simulink model "dsp_channelized_receiver_"  (R2021a)
settings: Solver=VariableStepAuto  StartTime=0.0  StopTime=sim_time  RelTol=1e-3
values from neighbouring files (symbols this model uses):
  sim_time = 1e-3    (= 0.001)    [rx_dsp_core_init_hw.m]
  ts = 1/fs    (= 2.5e-10)    [rx_dsp_core_init_hw.m]
undefined symbols (not defined in the file or in its folder): es1
libraries: xbsIndex_r4 x267, dspsrcs4 x3, simulink x1, dspswit3 x1
(part 2 of 2)

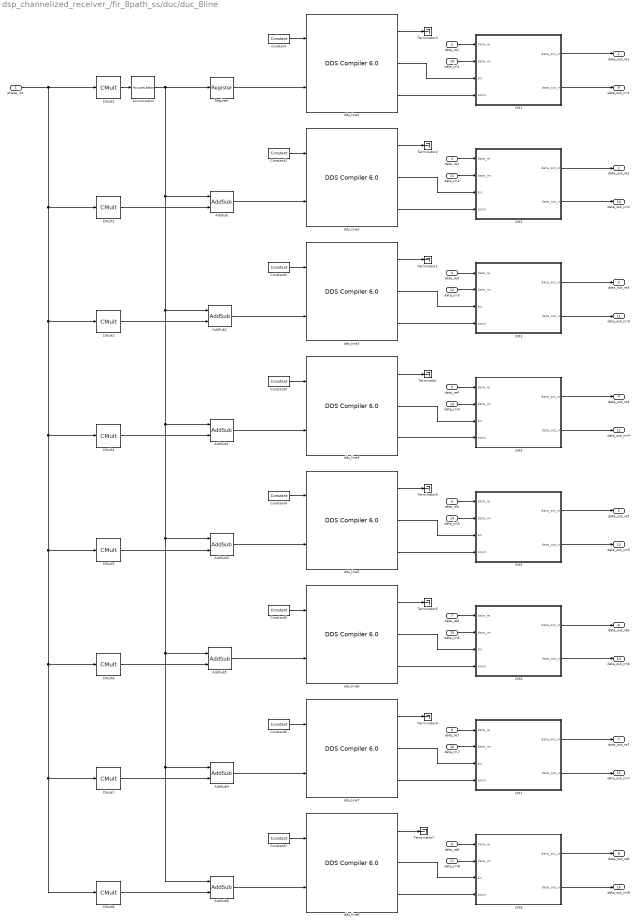
== system dsp_channelized_receiver_/fir_8path_ss/duc/duc_8line ==
  phase_inc : Inport
  data_re1 : Inport  Port=2
  data_re2 : Inport  Port=3
  data_re3 : Inport  Port=4
  data_re4 : Inport  Port=5
  data_re5 : Inport  Port=6
  data_re6 : Inport  Port=7
  data_re7 : Inport  Port=8
  data_re8 : Inport  Port=9
  data_im1 : Inport  Port=10
  data_im2 : Inport  Port=11
  data_im3 : Inport  Port=12
  data_im4 : Inport  Port=13
  data_im5 : Inport  Port=14
  data_im6 : Inport  Port=15
  data_im7 : Inport  Port=16
  data_im8 : Inport  Port=17
  Accumulator : xbsIndex_r4/Accumulator  operation=Add  n_bits=ddc_phase_width  overflow=Wrap  scale=1  rst=off  hasbypass=off  infoeditControl=reset for floating point data type must be asserted for a minimum of 2 cycles  en=off  latency=1  msb_inp=100  msb=100  lsb=-100  use_behavioral_HDL=on  implementation=Fabric  dbl_ovrd=off  block_type=accum
  AddSub{,1..6} (7 alike) : xbsIndex_r4/AddSub  mode=Addition  use_carryin=off  use_carryout=off  en=off  latency=1  precision=User Defined  arith_type=Unsigned  n_bits=ddc_phase_width  bin_pt=ddc_phase_width  quantization="Round  (unbiased: +/- Inf)"  overflow=Wrap  use_behavioral_HDL=off  hw_selection=Fabric  pipelined=off  dbl_ovrd=off  block_type=addsub
  CM1 : Subsystem
  CM2 : Subsystem
  CM3 : Subsystem
  CM4 : Subsystem
  CM5 : Subsystem
  CM6 : Subsystem
  CM7 : Subsystem
  CM8 : Subsystem
  CMult1 : xbsIndex_r4/CMult  const=1  gui_display_data_type=Fixed-point  const_n_bits=4  const_bin_pt=0  float_type=Single  exp_bits=8  fraction_bits=24  en=off  latency=1  precision=User Defined  arith_type=Unsigned  n_bits=ddc_phase_width  bin_pt=ddc_phase_width  quantization="Round  (unbiased: +/- Inf)"  overflow=Wrap  use_behavioral_HDL=off  mem_type=Distributed RAM  pipeline=off  dbl_ovrd=off  block_type=cmult
  CMult2 : xbsIndex_r4/CMult  const=2  gui_display_data_type=Fixed-point  const_n_bits=4  const_bin_pt=0  float_type=Single  exp_bits=8  fraction_bits=24  en=off  latency=1  precision=User Defined  arith_type=Unsigned  n_bits=ddc_phase_width  bin_pt=ddc_phase_width  quantization="Round  (unbiased: +/- Inf)"  overflow=Wrap  use_behavioral_HDL=off  mem_type=Distributed RAM  pipeline=off  dbl_ovrd=off  block_type=cmult
  CMult3 : xbsIndex_r4/CMult  const=8  gui_display_data_type=Fixed-point  const_n_bits=4  const_bin_pt=0  float_type=Single  exp_bits=8  fraction_bits=24  en=off  latency=1  precision=User Defined  arith_type=Unsigned  n_bits=ddc_phase_width  bin_pt=ddc_phase_width  quantization="Round  (unbiased: +/- Inf)"  overflow=Wrap  use_behavioral_HDL=off  mem_type=Distributed RAM  pipeline=off  dbl_ovrd=off  block_type=cmult
  CMult4 : xbsIndex_r4/CMult  const=3  gui_display_data_type=Fixed-point  const_n_bits=4  const_bin_pt=0  float_type=Single  exp_bits=8  fraction_bits=24  en=off  latency=1  precision=User Defined  arith_type=Unsigned  n_bits=ddc_phase_width  bin_pt=ddc_phase_width  quantization="Round  (unbiased: +/- Inf)"  overflow=Wrap  use_behavioral_HDL=off  mem_type=Distributed RAM  pipeline=off  dbl_ovrd=off  block_type=cmult
  CMult5 : xbsIndex_r4/CMult  const=4  gui_display_data_type=Fixed-point  const_n_bits=4  const_bin_pt=0  float_type=Single  exp_bits=8  fraction_bits=24  en=off  latency=1  precision=User Defined  arith_type=Unsigned  n_bits=ddc_phase_width  bin_pt=ddc_phase_width  quantization="Round  (unbiased: +/- Inf)"  overflow=Wrap  use_behavioral_HDL=off  mem_type=Distributed RAM  pipeline=off  dbl_ovrd=off  block_type=cmult
  CMult6 : xbsIndex_r4/CMult  const=5  gui_display_data_type=Fixed-point  const_n_bits=4  const_bin_pt=0  float_type=Single  exp_bits=8  fraction_bits=24  en=off  latency=1  precision=User Defined  arith_type=Unsigned  n_bits=ddc_phase_width  bin_pt=ddc_phase_width  quantization="Round  (unbiased: +/- Inf)"  overflow=Wrap  use_behavioral_HDL=off  mem_type=Distributed RAM  pipeline=off  dbl_ovrd=off  block_type=cmult
  CMult7 : xbsIndex_r4/CMult  const=6  gui_display_data_type=Fixed-point  const_n_bits=4  const_bin_pt=0  float_type=Single  exp_bits=8  fraction_bits=24  en=off  latency=1  precision=User Defined  arith_type=Unsigned  n_bits=ddc_phase_width  bin_pt=ddc_phase_width  quantization="Round  (unbiased: +/- Inf)"  overflow=Wrap  use_behavioral_HDL=off  mem_type=Distributed RAM  pipeline=off  dbl_ovrd=off  block_type=cmult
  CMult8 : xbsIndex_r4/CMult  const=7  gui_display_data_type=Fixed-point  const_n_bits=4  const_bin_pt=0  float_type=Single  exp_bits=8  fraction_bits=24  en=off  latency=1  precision=User Defined  arith_type=Unsigned  n_bits=ddc_phase_width  bin_pt=ddc_phase_width  quantization="Round  (unbiased: +/- Inf)"  overflow=Wrap  use_behavioral_HDL=off  mem_type=Distributed RAM  pipeline=off  dbl_ovrd=off  block_type=cmult
  Constant{,1..7} (8 alike) : xbsIndex_r4/Constant  const=1  gui_display_data_type=Boolean  arith_type=Boolean  n_bits=16  bin_pt=14  preci_type=Single  exp_width=8  frac_width=24  explicit_period=on  period=ts  equ=P=C  opselect=C  inp2=PCIN>>17  opr=+  inp1=P  carry=CIN  dbl_ovrd=off  block_type=constant
  Register : xbsIndex_r4/Register  init=0  rst=off  en=off  dbl_ovrd=off  block_type=register
  Terminator{,1..7} (8 alike) : Terminator
  dds_line{1..8} (8 alike) : xbsIndex_r4/DDS Compiler 6.0   partspresent=SIN_COS_LUT_only  dds_clock_rate=100  channels=1  mode_of_operation=Standard  modulus=9  parameter_entry=System_Parameters  spurious_free_dynamic_range=36.00000000  frequency_resolution=0.40000000  noise_shaping=None  phase_width=ddc_phase_width  output_width=ddc_data_width  output_selection=Sine_and_Cosine  negative_sine=off  negative_cosine=off  amplitude_mode=Full_Range  memory_type=Auto  optimization_goal=Auto  dsp48_use=Minimal  resync=off  latency_configuration=Auto  latency=1  has_phase_out=off  has_aclken=off  has_aresetn=off  explicit_period=off  period=1  data_has_tlast=Not_Required  has_tready=off  s_phase_has_tuser=Not_Required  m_data_has_tuser=Not_Required  m_phase_has_tuser=Not_Required  s_phase_tuser_width=1  output_form=Twos_Complement  s_config_sync_mode=On_Vector  phase_increment=Fixed  output_frequency1=0  output_frequency2=0  output_frequency3=0  output_frequency4=0  output_frequency5=0  output_frequency6=0  output_frequency7=0  output_frequency8=0  output_frequency9=0  output_frequency10=0  output_frequency11=0  output_frequency12=0  output_frequency13=0  output_frequency14=0  output_frequency15=0  output_frequency16=0  pinc1='0'  pinc2='0'  pinc3='0'  pinc4='0'  pinc5='0'  pinc6='0'  pinc7='0'  pinc8='0'  pinc9='0'  pinc10='0'  pinc11='0'  pinc12='0'  pinc13='0'  pinc14='0'  pinc15='0'  pinc16='0'  phase_offset=None  phase_offset_angles1=0  phase_offset_angles2=0  phase_offset_angles3=0  phase_offset_angles4=0  phase_offset_angles5=0  phase_offset_angles6=0  phase_offset_angles7=0  phase_offset_angles8=0  phase_offset_angles9=0  phase_offset_angles10=0  phase_offset_angles11=0  phase_offset_angles12=0  phase_offset_angles13=0  phase_offset_angles14=0  phase_offset_angles15=0  phase_offset_angles16=0  poff1='0'  poff2='0'  poff3='0'  poff4='0'  poff5='0'  poff6='0'  poff7='0'  poff8='0'  poff9='0'  poff10='0'  poff11='0'  poff12='0'  poff13='0'  poff14='0'  poff15='0'  poff16='0'  trim_axipin_name=on  simulation_type=hybrid_sim  simulation_model=sysgen:xddsv6_0_cmodel  data_path_portlist={ 's_axis_config_tdata_poff', 's_axis_config_tdata_chan0_poff', 's_axis_config_tdata_pinc', 's_axis_config_tdata_chan0_pinc', 's_axis_phase_tdata_resync', 's_axis_phase_tdata_chan0_resync', 's_axis_phase_tdata_poff', 's_axis_phase_tdata_chan0_poff', 's_axis_phase_tdata_pinc', 's_axis_phase_tdata_chan0_pinc', 's_axis_phase_tdata_phase_in', 'm_axis_data_tdata_sine', 'm_axis_data_tdata_chan0_sine', 'm_axis_data_tdata_cosine', 'm_axis_data_tdata_chan0_cosine', 'm_axis_phase_tdata_phase_out', 'm_axis_phase_tdata_chan0_phase_out'}  por_mode=false  gui_behaviour=Sysgen  ip_name=DDS Compiler  ip_version=6.0  dsptool_ready=true  wrapper_available=true  port_translation_map={ 'aclken' => 'en', 'aresetn' => 'rst' }  ipcore_usecache=true  ipcore_useipmodelcache=true  ipcore_xco_need_fpga_part=true  ipcore_verbose=false  block_type=dds_compiler_v6_0
  data_out_re1 : Outport
  data_out_re2 : Outport  Port=2
  data_out_re3 : Outport  Port=3
  data_out_re4 : Outport  Port=4
  data_out_re5 : Outport  Port=5
  data_out_re6 : Outport  Port=6
  data_out_re7 : Outport  Port=7
  data_out_re8 : Outport  Port=8
  data_out_im1 : Outport  Port=9
  data_out_im2 : Outport  Port=10
  data_out_im3 : Outport  Port=11
  data_out_im4 : Outport  Port=12
  data_out_im5 : Outport  Port=13
  data_out_im6 : Outport  Port=14
  data_out_im7 : Outport  Port=15
  data_out_im8 : Outport  Port=16
  wires:
  Register/1 -> dds_line1/2
  CMult3/1 -> Accumulator/1
  AddSub2/1 -> dds_line3/2
  AddSub1/1 -> dds_line4/2
  AddSub/1 -> dds_line2/2
  dds_line3/1 -> Terminator1/1
  Constant/1 -> dds_line1/1
  dds_line1/1 -> Terminator3/1
  Constant1/1 -> dds_line2/1
  Constant2/1 -> dds_line3/1
  dds_line2/1 -> Terminator2/1
  dds_line4/1 -> Terminator/1
  Constant3/1 -> dds_line4/1
  Constant6/1 -> dds_line7/1
  dds_line7/1 -> Terminator4/1
  dds_line5/1 -> Terminator6/1
  Constant5/1 -> dds_line6/1
  Constant4/1 -> dds_line5/1
  dds_line6/1 -> Terminator5/1
  AddSub3/1 -> dds_line5/2
  AddSub4/1 -> dds_line7/2
  AddSub5/1 -> dds_line6/2
  CMult1/1 -> AddSub/2
  CMult2/1 -> AddSub2/2
  CMult4/1 -> AddSub1/2
  CMult5/1 -> AddSub3/2
  CMult6/1 -> AddSub5/2
  CMult7/1 -> AddSub4/2
  CMult8/1 -> AddSub6/2
  phase_inc/1 -> CMult8/1, CMult7/1, CMult6/1, CMult5/1, CMult4/1, CMult2/1, CMult1/1, CMult3/1
  Accumulator/1 -> AddSub6/1, AddSub4/1, AddSub5/1, AddSub3/1, AddSub1/1, AddSub2/1, AddSub/1, Register/1
  AddSub6/1 -> dds_line8/2
  dds_line8/1 -> Terminator7/1
  Constant7/1 -> dds_line8/1
  dds_line1/3 -> CM1/4(cosin)
  dds_line1/2 -> CM1/3(sin)
  dds_line2/3 -> CM2/4(cosin)
  dds_line3/3 -> CM3/4(cosin)
  dds_line4/3 -> CM4/4(cosin)
  dds_line4/2 -> CM4/3(sin)
  dds_line3/2 -> CM3/3(sin)
  dds_line2/2 -> CM2/3(sin)
  dds_line5/3 -> CM5/4(cosin)
  dds_line5/2 -> CM5/3(sin)
  dds_line6/3 -> CM6/4(cosin)
  dds_line6/2 -> CM6/3(sin)
  dds_line7/3 -> CM7/4(cosin)
  dds_line7/2 -> CM7/3(sin)
  dds_line8/3 -> CM8/4(cosin)
  dds_line8/2 -> CM8/3(sin)
  data_re1/1 -> CM1/1(data_re)
  data_re2/1 -> CM2/1(data_re)
  data_re3/1 -> CM3/1(data_re)
  data_re4/1 -> CM4/1(data_re)
  data_re5/1 -> CM5/1(data_re)
  data_re6/1 -> CM6/1(data_re)
  data_re7/1 -> CM7/1(data_re)
  data_re8/1 -> CM8/1(data_re)
  data_im1/1 -> CM1/2(data_im)
  data_im2/1 -> CM2/2(data_im)
  data_im3/1 -> CM3/2(data_im)
  data_im4/1 -> CM4/2(data_im)
  data_im5/1 -> CM5/2(data_im)
  data_im6/1 -> CM6/2(data_im)
  data_im7/1 -> CM7/2(data_im)
  data_im8/1 -> CM8/2(data_im)
  CM1/1(data_out_im) -> data_out_re1/1
  CM1/2(data_out_re) -> data_out_im1/1
  CM2/2(data_out_re) -> data_out_im2/1
  CM2/1(data_out_im) -> data_out_re2/1
  CM3/2(data_out_re) -> data_out_im3/1
  CM3/1(data_out_im) -> data_out_re3/1
  CM4/2(data_out_re) -> data_out_im4/1
  CM4/1(data_out_im) -> data_out_re4/1
  CM5/2(data_out_re) -> data_out_im5/1
  CM5/1(data_out_im) -> data_out_re5/1
  CM6/2(data_out_re) -> data_out_im6/1
  CM6/1(data_out_im) -> data_out_re6/1
  CM7/2(data_out_re) -> data_out_im7/1
  CM7/1(data_out_im) -> data_out_re7/1
  CM8/2(data_out_re) -> data_out_im8/1
  CM8/1(data_out_im) -> data_out_re8/1

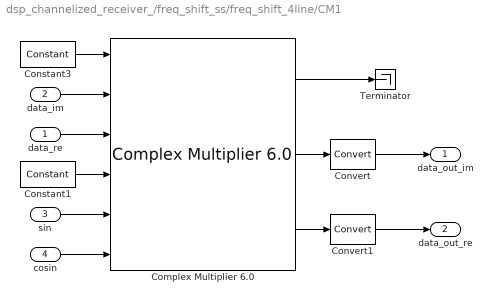
== system dsp_channelized_receiver_/freq_shift_ss/freq_shift_4line/CM1 ==
  data_re : Inport
  data_im : Inport  Port=2
  sin : Inport  Port=3
  cosin : Inport  Port=4
  Complex Multiplier 6.0 : xbsIndex_r4/Complex Multiplier 6.0   hasatlast=off  hasatuser=off  atuserwidth=1  hasbtlast=off  hasbtuser=off  btuserwidth=1  multtype=Use_Mults  optimizegoal=Performance  flowcontrol=NonBlocking  outputwidth=33  roundmode=Truncate  hasctrltlast=off  hasctrltuser=off  ctrltuserwidth=1  outtlastbehv=Null  latencyconfig=Automatic  minimumlatency=34  aclken=off  aresetn=off  trim_axipin_name=on  simulation_type=hybrid_sim  simulation_model=sysgen:cmpy_v6_0  data_path_portlist={ 's_axis_a_tdata_real', 's_axis_a_tdata_imag', 's_axis_b_tdata_real', 's_axis_b_tdata_imag', 's_axis_ctrl_tdata_rounding_bit', 'm_axis_dout_tdata_real', 'm_axis_dout_tdata_imag' }  aportwidth=63  bportwidth=63  ip_name=Complex Multiplier  ip_version=6.0  dsptool_ready=true  ipcore_usecache=true  ipcore_useipmodelcache=true  ipcore_verbose=false  ipcore_latency_parameter='minimumlatency'  wrapper_available=true  port_translation_map={ 'aclken' => 'en', 'aresetn' => 'rst'}  block_type=cmpy_v6_0
  Constant1 : xbsIndex_r4/Constant  const=1  gui_display_data_type=Boolean  arith_type=Boolean  n_bits=16  bin_pt=14  preci_type=Single  exp_width=8  frac_width=24  explicit_period=on  period=ts*4  equ=P=C  opselect=C  inp2=PCIN>>17  opr=+  inp1=P  carry=CIN  dbl_ovrd=off  block_type=constant
  Constant3 : xbsIndex_r4/Constant  const=1  gui_display_data_type=Boolean  arith_type=Boolean  n_bits=16  bin_pt=14  preci_type=Single  exp_width=8  frac_width=24  explicit_period=on  period=ts*4  equ=P=C  opselect=C  inp2=PCIN>>17  opr=+  inp1=P  carry=CIN  dbl_ovrd=off  block_type=constant
  Convert : xbsIndex_r4/Convert  gui_display_data_type=Fixed-point  arith_type="Signed  (2's comp)"  n_bits=16  bin_pt=0  float_type=Single  exp_bits=8  fraction_bits=24  quantization="Round  (unbiased: +/- Inf)"  overflow=Saturate  en=off  latency=1  pipeline=off  dbl_ovrd=off  block_type=convert
  Convert1 : xbsIndex_r4/Convert  gui_display_data_type=Fixed-point  arith_type="Signed  (2's comp)"  n_bits=16  bin_pt=0  float_type=Single  exp_bits=8  fraction_bits=24  quantization="Round  (unbiased: +/- Inf)"  overflow=Saturate  en=off  latency=1  pipeline=off  dbl_ovrd=off  block_type=convert
  Terminator : Terminator
  data_out_im : Outport
  data_out_re : Outport  Port=2
  wires:
  Convert/1 -> data_out_im/1
  Convert1/1 -> data_out_re/1
  data_re/1 -> Complex Multiplier 6.0/3
  Constant3/1 -> Complex Multiplier 6.0/1
  Complex Multiplier 6.0/2 -> Convert/1
  Complex Multiplier 6.0/1 -> Terminator/1
  Constant1/1 -> Complex Multiplier 6.0/4
  sin/1 -> Complex Multiplier 6.0/5
  cosin/1 -> Complex Multiplier 6.0/6
  data_im/1 -> Complex Multiplier 6.0/2
  Complex Multiplier 6.0/3 -> Convert1/1

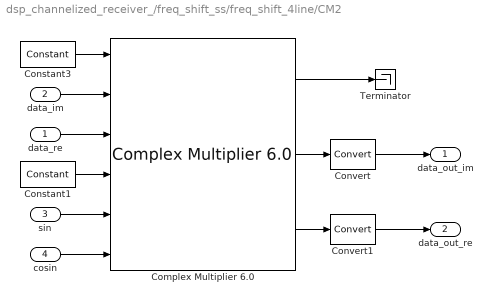
== system dsp_channelized_receiver_/freq_shift_ss/freq_shift_4line/CM2 ==
  data_re : Inport
  data_im : Inport  Port=2
  sin : Inport  Port=3
  cosin : Inport  Port=4
  Complex Multiplier 6.0 : xbsIndex_r4/Complex Multiplier 6.0   hasatlast=off  hasatuser=off  atuserwidth=1  hasbtlast=off  hasbtuser=off  btuserwidth=1  multtype=Use_Mults  optimizegoal=Performance  flowcontrol=NonBlocking  outputwidth=33  roundmode=Truncate  hasctrltlast=off  hasctrltuser=off  ctrltuserwidth=1  outtlastbehv=Null  latencyconfig=Automatic  minimumlatency=34  aclken=off  aresetn=off  trim_axipin_name=on  simulation_type=hybrid_sim  simulation_model=sysgen:cmpy_v6_0  data_path_portlist={ 's_axis_a_tdata_real', 's_axis_a_tdata_imag', 's_axis_b_tdata_real', 's_axis_b_tdata_imag', 's_axis_ctrl_tdata_rounding_bit', 'm_axis_dout_tdata_real', 'm_axis_dout_tdata_imag' }  aportwidth=63  bportwidth=63  ip_name=Complex Multiplier  ip_version=6.0  dsptool_ready=true  ipcore_usecache=true  ipcore_useipmodelcache=true  ipcore_verbose=false  ipcore_latency_parameter='minimumlatency'  wrapper_available=true  port_translation_map={ 'aclken' => 'en', 'aresetn' => 'rst'}  block_type=cmpy_v6_0
  Constant1 : xbsIndex_r4/Constant  const=1  gui_display_data_type=Boolean  arith_type=Boolean  n_bits=16  bin_pt=14  preci_type=Single  exp_width=8  frac_width=24  explicit_period=on  period=ts*4  equ=P=C  opselect=C  inp2=PCIN>>17  opr=+  inp1=P  carry=CIN  dbl_ovrd=off  block_type=constant
  Constant3 : xbsIndex_r4/Constant  const=1  gui_display_data_type=Boolean  arith_type=Boolean  n_bits=16  bin_pt=14  preci_type=Single  exp_width=8  frac_width=24  explicit_period=on  period=ts*4  equ=P=C  opselect=C  inp2=PCIN>>17  opr=+  inp1=P  carry=CIN  dbl_ovrd=off  block_type=constant
  Convert : xbsIndex_r4/Convert  gui_display_data_type=Fixed-point  arith_type="Signed  (2's comp)"  n_bits=16  bin_pt=0  float_type=Single  exp_bits=8  fraction_bits=24  quantization="Round  (unbiased: +/- Inf)"  overflow=Saturate  en=off  latency=1  pipeline=off  dbl_ovrd=off  block_type=convert
  Convert1 : xbsIndex_r4/Convert  gui_display_data_type=Fixed-point  arith_type="Signed  (2's comp)"  n_bits=16  bin_pt=0  float_type=Single  exp_bits=8  fraction_bits=24  quantization="Round  (unbiased: +/- Inf)"  overflow=Saturate  en=off  latency=1  pipeline=off  dbl_ovrd=off  block_type=convert
  Terminator : Terminator
  data_out_im : Outport
  data_out_re : Outport  Port=2
  wires:
  Complex Multiplier 6.0/3 -> Convert1/1
  data_im/1 -> Complex Multiplier 6.0/2
  cosin/1 -> Complex Multiplier 6.0/6
  sin/1 -> Complex Multiplier 6.0/5
  Constant1/1 -> Complex Multiplier 6.0/4
  Complex Multiplier 6.0/1 -> Terminator/1
  Complex Multiplier 6.0/2 -> Convert/1
  Constant3/1 -> Complex Multiplier 6.0/1
  data_re/1 -> Complex Multiplier 6.0/3
  Convert1/1 -> data_out_re/1
  Convert/1 -> data_out_im/1

== system dsp_channelized_receiver_/freq_shift_ss/freq_shift_4line/CM3 ==
  data_re : Inport
  data_im : Inport  Port=2
  sin : Inport  Port=3
  cosin : Inport  Port=4
  Complex Multiplier 6.0 : xbsIndex_r4/Complex Multiplier 6.0   hasatlast=off  hasatuser=off  atuserwidth=1  hasbtlast=off  hasbtuser=off  btuserwidth=1  multtype=Use_Mults  optimizegoal=Performance  flowcontrol=NonBlocking  outputwidth=33  roundmode=Truncate  hasctrltlast=off  hasctrltuser=off  ctrltuserwidth=1  outtlastbehv=Null  latencyconfig=Automatic  minimumlatency=34  aclken=off  aresetn=off  trim_axipin_name=on  simulation_type=hybrid_sim  simulation_model=sysgen:cmpy_v6_0  data_path_portlist={ 's_axis_a_tdata_real', 's_axis_a_tdata_imag', 's_axis_b_tdata_real', 's_axis_b_tdata_imag', 's_axis_ctrl_tdata_rounding_bit', 'm_axis_dout_tdata_real', 'm_axis_dout_tdata_imag' }  aportwidth=63  bportwidth=63  ip_name=Complex Multiplier  ip_version=6.0  dsptool_ready=true  ipcore_usecache=true  ipcore_useipmodelcache=true  ipcore_verbose=false  ipcore_latency_parameter='minimumlatency'  wrapper_available=true  port_translation_map={ 'aclken' => 'en', 'aresetn' => 'rst'}  block_type=cmpy_v6_0
  Constant1 : xbsIndex_r4/Constant  const=1  gui_display_data_type=Boolean  arith_type=Boolean  n_bits=16  bin_pt=14  preci_type=Single  exp_width=8  frac_width=24  explicit_period=on  period=ts*4  equ=P=C  opselect=C  inp2=PCIN>>17  opr=+  inp1=P  carry=CIN  dbl_ovrd=off  block_type=constant
  Constant3 : xbsIndex_r4/Constant  const=1  gui_display_data_type=Boolean  arith_type=Boolean  n_bits=16  bin_pt=14  preci_type=Single  exp_width=8  frac_width=24  explicit_period=on  period=ts*4  equ=P=C  opselect=C  inp2=PCIN>>17  opr=+  inp1=P  carry=CIN  dbl_ovrd=off  block_type=constant
  Convert : xbsIndex_r4/Convert  gui_display_data_type=Fixed-point  arith_type="Signed  (2's comp)"  n_bits=16  bin_pt=0  float_type=Single  exp_bits=8  fraction_bits=24  quantization="Round  (unbiased: +/- Inf)"  overflow=Saturate  en=off  latency=1  pipeline=off  dbl_ovrd=off  block_type=convert
  Convert1 : xbsIndex_r4/Convert  gui_display_data_type=Fixed-point  arith_type="Signed  (2's comp)"  n_bits=16  bin_pt=0  float_type=Single  exp_bits=8  fraction_bits=24  quantization="Round  (unbiased: +/- Inf)"  overflow=Saturate  en=off  latency=1  pipeline=off  dbl_ovrd=off  block_type=convert
  Terminator : Terminator
  data_out_im : Outport
  data_out_re : Outport  Port=2
  wires:
  Convert/1 -> data_out_im/1
  Convert1/1 -> data_out_re/1
  data_re/1 -> Complex Multiplier 6.0/3
  Constant3/1 -> Complex Multiplier 6.0/1
  Complex Multiplier 6.0/2 -> Convert/1
  Complex Multiplier 6.0/1 -> Terminator/1
  Constant1/1 -> Complex Multiplier 6.0/4
  sin/1 -> Complex Multiplier 6.0/5
  cosin/1 -> Complex Multiplier 6.0/6
  data_im/1 -> Complex Multiplier 6.0/2
  Complex Multiplier 6.0/3 -> Convert1/1

== system dsp_channelized_receiver_/freq_shift_ss/freq_shift_4line/CM4 ==
  data_re : Inport
  data_im : Inport  Port=2
  sin : Inport  Port=3
  cosin : Inport  Port=4
  Complex Multiplier 6.0 : xbsIndex_r4/Complex Multiplier 6.0   hasatlast=off  hasatuser=off  atuserwidth=1  hasbtlast=off  hasbtuser=off  btuserwidth=1  multtype=Use_Mults  optimizegoal=Performance  flowcontrol=NonBlocking  outputwidth=33  roundmode=Truncate  hasctrltlast=off  hasctrltuser=off  ctrltuserwidth=1  outtlastbehv=Null  latencyconfig=Automatic  minimumlatency=34  aclken=off  aresetn=off  trim_axipin_name=on  simulation_type=hybrid_sim  simulation_model=sysgen:cmpy_v6_0  data_path_portlist={ 's_axis_a_tdata_real', 's_axis_a_tdata_imag', 's_axis_b_tdata_real', 's_axis_b_tdata_imag', 's_axis_ctrl_tdata_rounding_bit', 'm_axis_dout_tdata_real', 'm_axis_dout_tdata_imag' }  aportwidth=63  bportwidth=63  ip_name=Complex Multiplier  ip_version=6.0  dsptool_ready=true  ipcore_usecache=true  ipcore_useipmodelcache=true  ipcore_verbose=false  ipcore_latency_parameter='minimumlatency'  wrapper_available=true  port_translation_map={ 'aclken' => 'en', 'aresetn' => 'rst'}  block_type=cmpy_v6_0
  Constant1 : xbsIndex_r4/Constant  const=1  gui_display_data_type=Boolean  arith_type=Boolean  n_bits=16  bin_pt=14  preci_type=Single  exp_width=8  frac_width=24  explicit_period=on  period=ts*4  equ=P=C  opselect=C  inp2=PCIN>>17  opr=+  inp1=P  carry=CIN  dbl_ovrd=off  block_type=constant
  Constant3 : xbsIndex_r4/Constant  const=1  gui_display_data_type=Boolean  arith_type=Boolean  n_bits=16  bin_pt=14  preci_type=Single  exp_width=8  frac_width=24  explicit_period=on  period=ts*4  equ=P=C  opselect=C  inp2=PCIN>>17  opr=+  inp1=P  carry=CIN  dbl_ovrd=off  block_type=constant
  Convert : xbsIndex_r4/Convert  gui_display_data_type=Fixed-point  arith_type="Signed  (2's comp)"  n_bits=16  bin_pt=0  float_type=Single  exp_bits=8  fraction_bits=24  quantization="Round  (unbiased: +/- Inf)"  overflow=Saturate  en=off  latency=1  pipeline=off  dbl_ovrd=off  block_type=convert
  Convert1 : xbsIndex_r4/Convert  gui_display_data_type=Fixed-point  arith_type="Signed  (2's comp)"  n_bits=16  bin_pt=0  float_type=Single  exp_bits=8  fraction_bits=24  quantization="Round  (unbiased: +/- Inf)"  overflow=Saturate  en=off  latency=1  pipeline=off  dbl_ovrd=off  block_type=convert
  Terminator : Terminator
  data_out_im : Outport
  data_out_re : Outport  Port=2
  wires:
  Complex Multiplier 6.0/3 -> Convert1/1
  data_im/1 -> Complex Multiplier 6.0/2
  cosin/1 -> Complex Multiplier 6.0/6
  sin/1 -> Complex Multiplier 6.0/5
  Constant1/1 -> Complex Multiplier 6.0/4
  Complex Multiplier 6.0/1 -> Terminator/1
  Complex Multiplier 6.0/2 -> Convert/1
  Constant3/1 -> Complex Multiplier 6.0/1
  data_re/1 -> Complex Multiplier 6.0/3
  Convert1/1 -> data_out_re/1
  Convert/1 -> data_out_im/1

== system dsp_channelized_receiver_/fir_8path_ss/duc/duc_8line/CM1 ==
  data_re : Inport
  data_im : Inport  Port=2
  sin : Inport  Port=3
  cosin : Inport  Port=4
  Complex Multiplier 6.0 : xbsIndex_r4/Complex Multiplier 6.0   hasatlast=off  hasatuser=off  atuserwidth=1  hasbtlast=off  hasbtuser=off  btuserwidth=1  multtype=Use_Mults  optimizegoal=Performance  flowcontrol=NonBlocking  outputwidth=33  roundmode=Truncate  hasctrltlast=off  hasctrltuser=off  ctrltuserwidth=1  outtlastbehv=Null  latencyconfig=Automatic  minimumlatency=34  aclken=off  aresetn=off  trim_axipin_name=on  simulation_type=hybrid_sim  simulation_model=sysgen:cmpy_v6_0  data_path_portlist={ 's_axis_a_tdata_real', 's_axis_a_tdata_imag', 's_axis_b_tdata_real', 's_axis_b_tdata_imag', 's_axis_ctrl_tdata_rounding_bit', 'm_axis_dout_tdata_real', 'm_axis_dout_tdata_imag' }  aportwidth=63  bportwidth=63  ip_name=Complex Multiplier  ip_version=6.0  dsptool_ready=true  ipcore_usecache=true  ipcore_useipmodelcache=true  ipcore_verbose=false  ipcore_latency_parameter='minimumlatency'  wrapper_available=true  port_translation_map={ 'aclken' => 'en', 'aresetn' => 'rst'}  block_type=cmpy_v6_0
  Constant1 : xbsIndex_r4/Constant  const=1  gui_display_data_type=Boolean  arith_type=Boolean  n_bits=16  bin_pt=14  preci_type=Single  exp_width=8  frac_width=24  explicit_period=on  period=ts*4  equ=P=C  opselect=C  inp2=PCIN>>17  opr=+  inp1=P  carry=CIN  dbl_ovrd=off  block_type=constant
  Constant3 : xbsIndex_r4/Constant  const=1  gui_display_data_type=Boolean  arith_type=Boolean  n_bits=16  bin_pt=14  preci_type=Single  exp_width=8  frac_width=24  explicit_period=on  period=ts*4  equ=P=C  opselect=C  inp2=PCIN>>17  opr=+  inp1=P  carry=CIN  dbl_ovrd=off  block_type=constant
  Convert : xbsIndex_r4/Convert  gui_display_data_type=Fixed-point  arith_type="Signed  (2's comp)"  n_bits=16  bin_pt=0  float_type=Single  exp_bits=8  fraction_bits=24  quantization="Round  (unbiased: +/- Inf)"  overflow=Saturate  en=off  latency=1  pipeline=off  dbl_ovrd=off  block_type=convert
  Convert1 : xbsIndex_r4/Convert  gui_display_data_type=Fixed-point  arith_type="Signed  (2's comp)"  n_bits=16  bin_pt=0  float_type=Single  exp_bits=8  fraction_bits=24  quantization="Round  (unbiased: +/- Inf)"  overflow=Saturate  en=off  latency=1  pipeline=off  dbl_ovrd=off  block_type=convert
  Terminator : Terminator
  data_out_im : Outport
  data_out_re : Outport  Port=2
  wires:
  Complex Multiplier 6.0/3 -> Convert1/1
  data_im/1 -> Complex Multiplier 6.0/2
  cosin/1 -> Complex Multiplier 6.0/6
  sin/1 -> Complex Multiplier 6.0/5
  Constant1/1 -> Complex Multiplier 6.0/4
  Complex Multiplier 6.0/1 -> Terminator/1
  Complex Multiplier 6.0/2 -> Convert/1
  Constant3/1 -> Complex Multiplier 6.0/1
  data_re/1 -> Complex Multiplier 6.0/3
  Convert1/1 -> data_out_re/1
  Convert/1 -> data_out_im/1

== system dsp_channelized_receiver_/fir_8path_ss/duc/duc_8line/CM2 ==
  data_re : Inport
  data_im : Inport  Port=2
  sin : Inport  Port=3
  cosin : Inport  Port=4
  Complex Multiplier 6.0 : xbsIndex_r4/Complex Multiplier 6.0   hasatlast=off  hasatuser=off  atuserwidth=1  hasbtlast=off  hasbtuser=off  btuserwidth=1  multtype=Use_Mults  optimizegoal=Performance  flowcontrol=NonBlocking  outputwidth=33  roundmode=Truncate  hasctrltlast=off  hasctrltuser=off  ctrltuserwidth=1  outtlastbehv=Null  latencyconfig=Automatic  minimumlatency=34  aclken=off  aresetn=off  trim_axipin_name=on  simulation_type=hybrid_sim  simulation_model=sysgen:cmpy_v6_0  data_path_portlist={ 's_axis_a_tdata_real', 's_axis_a_tdata_imag', 's_axis_b_tdata_real', 's_axis_b_tdata_imag', 's_axis_ctrl_tdata_rounding_bit', 'm_axis_dout_tdata_real', 'm_axis_dout_tdata_imag' }  aportwidth=63  bportwidth=63  ip_name=Complex Multiplier  ip_version=6.0  dsptool_ready=true  ipcore_usecache=true  ipcore_useipmodelcache=true  ipcore_verbose=false  ipcore_latency_parameter='minimumlatency'  wrapper_available=true  port_translation_map={ 'aclken' => 'en', 'aresetn' => 'rst'}  block_type=cmpy_v6_0
  Constant1 : xbsIndex_r4/Constant  const=1  gui_display_data_type=Boolean  arith_type=Boolean  n_bits=16  bin_pt=14  preci_type=Single  exp_width=8  frac_width=24  explicit_period=on  period=ts*4  equ=P=C  opselect=C  inp2=PCIN>>17  opr=+  inp1=P  carry=CIN  dbl_ovrd=off  block_type=constant
  Constant3 : xbsIndex_r4/Constant  const=1  gui_display_data_type=Boolean  arith_type=Boolean  n_bits=16  bin_pt=14  preci_type=Single  exp_width=8  frac_width=24  explicit_period=on  period=ts*4  equ=P=C  opselect=C  inp2=PCIN>>17  opr=+  inp1=P  carry=CIN  dbl_ovrd=off  block_type=constant
  Convert : xbsIndex_r4/Convert  gui_display_data_type=Fixed-point  arith_type="Signed  (2's comp)"  n_bits=16  bin_pt=0  float_type=Single  exp_bits=8  fraction_bits=24  quantization="Round  (unbiased: +/- Inf)"  overflow=Saturate  en=off  latency=1  pipeline=off  dbl_ovrd=off  block_type=convert
  Convert1 : xbsIndex_r4/Convert  gui_display_data_type=Fixed-point  arith_type="Signed  (2's comp)"  n_bits=16  bin_pt=0  float_type=Single  exp_bits=8  fraction_bits=24  quantization="Round  (unbiased: +/- Inf)"  overflow=Saturate  en=off  latency=1  pipeline=off  dbl_ovrd=off  block_type=convert
  Terminator : Terminator
  data_out_im : Outport
  data_out_re : Outport  Port=2
  wires:
  Convert/1 -> data_out_im/1
  Convert1/1 -> data_out_re/1
  data_re/1 -> Complex Multiplier 6.0/3
  Constant3/1 -> Complex Multiplier 6.0/1
  Complex Multiplier 6.0/2 -> Convert/1
  Complex Multiplier 6.0/1 -> Terminator/1
  Constant1/1 -> Complex Multiplier 6.0/4
  sin/1 -> Complex Multiplier 6.0/5
  cosin/1 -> Complex Multiplier 6.0/6
  data_im/1 -> Complex Multiplier 6.0/2
  Complex Multiplier 6.0/3 -> Convert1/1

== system dsp_channelized_receiver_/fir_8path_ss/duc/duc_8line/CM3 ==
  data_re : Inport
  data_im : Inport  Port=2
  sin : Inport  Port=3
  cosin : Inport  Port=4
  Complex Multiplier 6.0 : xbsIndex_r4/Complex Multiplier 6.0   hasatlast=off  hasatuser=off  atuserwidth=1  hasbtlast=off  hasbtuser=off  btuserwidth=1  multtype=Use_Mults  optimizegoal=Performance  flowcontrol=NonBlocking  outputwidth=33  roundmode=Truncate  hasctrltlast=off  hasctrltuser=off  ctrltuserwidth=1  outtlastbehv=Null  latencyconfig=Automatic  minimumlatency=34  aclken=off  aresetn=off  trim_axipin_name=on  simulation_type=hybrid_sim  simulation_model=sysgen:cmpy_v6_0  data_path_portlist={ 's_axis_a_tdata_real', 's_axis_a_tdata_imag', 's_axis_b_tdata_real', 's_axis_b_tdata_imag', 's_axis_ctrl_tdata_rounding_bit', 'm_axis_dout_tdata_real', 'm_axis_dout_tdata_imag' }  aportwidth=63  bportwidth=63  ip_name=Complex Multiplier  ip_version=6.0  dsptool_ready=true  ipcore_usecache=true  ipcore_useipmodelcache=true  ipcore_verbose=false  ipcore_latency_parameter='minimumlatency'  wrapper_available=true  port_translation_map={ 'aclken' => 'en', 'aresetn' => 'rst'}  block_type=cmpy_v6_0
  Constant1 : xbsIndex_r4/Constant  const=1  gui_display_data_type=Boolean  arith_type=Boolean  n_bits=16  bin_pt=14  preci_type=Single  exp_width=8  frac_width=24  explicit_period=on  period=ts*4  equ=P=C  opselect=C  inp2=PCIN>>17  opr=+  inp1=P  carry=CIN  dbl_ovrd=off  block_type=constant
  Constant3 : xbsIndex_r4/Constant  const=1  gui_display_data_type=Boolean  arith_type=Boolean  n_bits=16  bin_pt=14  preci_type=Single  exp_width=8  frac_width=24  explicit_period=on  period=ts*4  equ=P=C  opselect=C  inp2=PCIN>>17  opr=+  inp1=P  carry=CIN  dbl_ovrd=off  block_type=constant
  Convert : xbsIndex_r4/Convert  gui_display_data_type=Fixed-point  arith_type="Signed  (2's comp)"  n_bits=16  bin_pt=0  float_type=Single  exp_bits=8  fraction_bits=24  quantization="Round  (unbiased: +/- Inf)"  overflow=Saturate  en=off  latency=1  pipeline=off  dbl_ovrd=off  block_type=convert
  Convert1 : xbsIndex_r4/Convert  gui_display_data_type=Fixed-point  arith_type="Signed  (2's comp)"  n_bits=16  bin_pt=0  float_type=Single  exp_bits=8  fraction_bits=24  quantization="Round  (unbiased: +/- Inf)"  overflow=Saturate  en=off  latency=1  pipeline=off  dbl_ovrd=off  block_type=convert
  Terminator : Terminator
  data_out_im : Outport
  data_out_re : Outport  Port=2
  wires:
  Complex Multiplier 6.0/3 -> Convert1/1
  data_im/1 -> Complex Multiplier 6.0/2
  cosin/1 -> Complex Multiplier 6.0/6
  sin/1 -> Complex Multiplier 6.0/5
  Constant1/1 -> Complex Multiplier 6.0/4
  Complex Multiplier 6.0/1 -> Terminator/1
  Complex Multiplier 6.0/2 -> Convert/1
  Constant3/1 -> Complex Multiplier 6.0/1
  data_re/1 -> Complex Multiplier 6.0/3
  Convert1/1 -> data_out_re/1
  Convert/1 -> data_out_im/1

== system dsp_channelized_receiver_/fir_8path_ss/duc/duc_8line/CM4 ==
  data_re : Inport
  data_im : Inport  Port=2
  sin : Inport  Port=3
  cosin : Inport  Port=4
  Complex Multiplier 6.0 : xbsIndex_r4/Complex Multiplier 6.0   hasatlast=off  hasatuser=off  atuserwidth=1  hasbtlast=off  hasbtuser=off  btuserwidth=1  multtype=Use_Mults  optimizegoal=Performance  flowcontrol=NonBlocking  outputwidth=33  roundmode=Truncate  hasctrltlast=off  hasctrltuser=off  ctrltuserwidth=1  outtlastbehv=Null  latencyconfig=Automatic  minimumlatency=34  aclken=off  aresetn=off  trim_axipin_name=on  simulation_type=hybrid_sim  simulation_model=sysgen:cmpy_v6_0  data_path_portlist={ 's_axis_a_tdata_real', 's_axis_a_tdata_imag', 's_axis_b_tdata_real', 's_axis_b_tdata_imag', 's_axis_ctrl_tdata_rounding_bit', 'm_axis_dout_tdata_real', 'm_axis_dout_tdata_imag' }  aportwidth=63  bportwidth=63  ip_name=Complex Multiplier  ip_version=6.0  dsptool_ready=true  ipcore_usecache=true  ipcore_useipmodelcache=true  ipcore_verbose=false  ipcore_latency_parameter='minimumlatency'  wrapper_available=true  port_translation_map={ 'aclken' => 'en', 'aresetn' => 'rst'}  block_type=cmpy_v6_0
  Constant1 : xbsIndex_r4/Constant  const=1  gui_display_data_type=Boolean  arith_type=Boolean  n_bits=16  bin_pt=14  preci_type=Single  exp_width=8  frac_width=24  explicit_period=on  period=ts*4  equ=P=C  opselect=C  inp2=PCIN>>17  opr=+  inp1=P  carry=CIN  dbl_ovrd=off  block_type=constant
  Constant3 : xbsIndex_r4/Constant  const=1  gui_display_data_type=Boolean  arith_type=Boolean  n_bits=16  bin_pt=14  preci_type=Single  exp_width=8  frac_width=24  explicit_period=on  period=ts*4  equ=P=C  opselect=C  inp2=PCIN>>17  opr=+  inp1=P  carry=CIN  dbl_ovrd=off  block_type=constant
  Convert : xbsIndex_r4/Convert  gui_display_data_type=Fixed-point  arith_type="Signed  (2's comp)"  n_bits=16  bin_pt=0  float_type=Single  exp_bits=8  fraction_bits=24  quantization="Round  (unbiased: +/- Inf)"  overflow=Saturate  en=off  latency=1  pipeline=off  dbl_ovrd=off  block_type=convert
  Convert1 : xbsIndex_r4/Convert  gui_display_data_type=Fixed-point  arith_type="Signed  (2's comp)"  n_bits=16  bin_pt=0  float_type=Single  exp_bits=8  fraction_bits=24  quantization="Round  (unbiased: +/- Inf)"  overflow=Saturate  en=off  latency=1  pipeline=off  dbl_ovrd=off  block_type=convert
  Terminator : Terminator
  data_out_im : Outport
  data_out_re : Outport  Port=2
  wires:
  Convert/1 -> data_out_im/1
  Convert1/1 -> data_out_re/1
  data_re/1 -> Complex Multiplier 6.0/3
  Constant3/1 -> Complex Multiplier 6.0/1
  Complex Multiplier 6.0/2 -> Convert/1
  Complex Multiplier 6.0/1 -> Terminator/1
  Constant1/1 -> Complex Multiplier 6.0/4
  sin/1 -> Complex Multiplier 6.0/5
  cosin/1 -> Complex Multiplier 6.0/6
  data_im/1 -> Complex Multiplier 6.0/2
  Complex Multiplier 6.0/3 -> Convert1/1

== system dsp_channelized_receiver_/fir_8path_ss/duc/duc_8line/CM5 ==
  data_re : Inport
  data_im : Inport  Port=2
  sin : Inport  Port=3
  cosin : Inport  Port=4
  Complex Multiplier 6.0 : xbsIndex_r4/Complex Multiplier 6.0   hasatlast=off  hasatuser=off  atuserwidth=1  hasbtlast=off  hasbtuser=off  btuserwidth=1  multtype=Use_Mults  optimizegoal=Performance  flowcontrol=NonBlocking  outputwidth=33  roundmode=Truncate  hasctrltlast=off  hasctrltuser=off  ctrltuserwidth=1  outtlastbehv=Null  latencyconfig=Automatic  minimumlatency=34  aclken=off  aresetn=off  trim_axipin_name=on  simulation_type=hybrid_sim  simulation_model=sysgen:cmpy_v6_0  data_path_portlist={ 's_axis_a_tdata_real', 's_axis_a_tdata_imag', 's_axis_b_tdata_real', 's_axis_b_tdata_imag', 's_axis_ctrl_tdata_rounding_bit', 'm_axis_dout_tdata_real', 'm_axis_dout_tdata_imag' }  aportwidth=63  bportwidth=63  ip_name=Complex Multiplier  ip_version=6.0  dsptool_ready=true  ipcore_usecache=true  ipcore_useipmodelcache=true  ipcore_verbose=false  ipcore_latency_parameter='minimumlatency'  wrapper_available=true  port_translation_map={ 'aclken' => 'en', 'aresetn' => 'rst'}  block_type=cmpy_v6_0
  Constant1 : xbsIndex_r4/Constant  const=1  gui_display_data_type=Boolean  arith_type=Boolean  n_bits=16  bin_pt=14  preci_type=Single  exp_width=8  frac_width=24  explicit_period=on  period=ts*4  equ=P=C  opselect=C  inp2=PCIN>>17  opr=+  inp1=P  carry=CIN  dbl_ovrd=off  block_type=constant
  Constant3 : xbsIndex_r4/Constant  const=1  gui_display_data_type=Boolean  arith_type=Boolean  n_bits=16  bin_pt=14  preci_type=Single  exp_width=8  frac_width=24  explicit_period=on  period=ts*4  equ=P=C  opselect=C  inp2=PCIN>>17  opr=+  inp1=P  carry=CIN  dbl_ovrd=off  block_type=constant
  Convert : xbsIndex_r4/Convert  gui_display_data_type=Fixed-point  arith_type="Signed  (2's comp)"  n_bits=16  bin_pt=0  float_type=Single  exp_bits=8  fraction_bits=24  quantization="Round  (unbiased: +/- Inf)"  overflow=Saturate  en=off  latency=1  pipeline=off  dbl_ovrd=off  block_type=convert
  Convert1 : xbsIndex_r4/Convert  gui_display_data_type=Fixed-point  arith_type="Signed  (2's comp)"  n_bits=16  bin_pt=0  float_type=Single  exp_bits=8  fraction_bits=24  quantization="Round  (unbiased: +/- Inf)"  overflow=Saturate  en=off  latency=1  pipeline=off  dbl_ovrd=off  block_type=convert
  Terminator : Terminator
  data_out_im : Outport
  data_out_re : Outport  Port=2
  wires:
  Complex Multiplier 6.0/3 -> Convert1/1
  data_im/1 -> Complex Multiplier 6.0/2
  cosin/1 -> Complex Multiplier 6.0/6
  sin/1 -> Complex Multiplier 6.0/5
  Constant1/1 -> Complex Multiplier 6.0/4
  Complex Multiplier 6.0/1 -> Terminator/1
  Complex Multiplier 6.0/2 -> Convert/1
  Constant3/1 -> Complex Multiplier 6.0/1
  data_re/1 -> Complex Multiplier 6.0/3
  Convert1/1 -> data_out_re/1
  Convert/1 -> data_out_im/1

== system dsp_channelized_receiver_/fir_8path_ss/duc/duc_8line/CM6 ==
  data_re : Inport
  data_im : Inport  Port=2
  sin : Inport  Port=3
  cosin : Inport  Port=4
  Complex Multiplier 6.0 : xbsIndex_r4/Complex Multiplier 6.0   hasatlast=off  hasatuser=off  atuserwidth=1  hasbtlast=off  hasbtuser=off  btuserwidth=1  multtype=Use_Mults  optimizegoal=Performance  flowcontrol=NonBlocking  outputwidth=33  roundmode=Truncate  hasctrltlast=off  hasctrltuser=off  ctrltuserwidth=1  outtlastbehv=Null  latencyconfig=Automatic  minimumlatency=34  aclken=off  aresetn=off  trim_axipin_name=on  simulation_type=hybrid_sim  simulation_model=sysgen:cmpy_v6_0  data_path_portlist={ 's_axis_a_tdata_real', 's_axis_a_tdata_imag', 's_axis_b_tdata_real', 's_axis_b_tdata_imag', 's_axis_ctrl_tdata_rounding_bit', 'm_axis_dout_tdata_real', 'm_axis_dout_tdata_imag' }  aportwidth=63  bportwidth=63  ip_name=Complex Multiplier  ip_version=6.0  dsptool_ready=true  ipcore_usecache=true  ipcore_useipmodelcache=true  ipcore_verbose=false  ipcore_latency_parameter='minimumlatency'  wrapper_available=true  port_translation_map={ 'aclken' => 'en', 'aresetn' => 'rst'}  block_type=cmpy_v6_0
  Constant1 : xbsIndex_r4/Constant  const=1  gui_display_data_type=Boolean  arith_type=Boolean  n_bits=16  bin_pt=14  preci_type=Single  exp_width=8  frac_width=24  explicit_period=on  period=ts*4  equ=P=C  opselect=C  inp2=PCIN>>17  opr=+  inp1=P  carry=CIN  dbl_ovrd=off  block_type=constant
  Constant3 : xbsIndex_r4/Constant  const=1  gui_display_data_type=Boolean  arith_type=Boolean  n_bits=16  bin_pt=14  preci_type=Single  exp_width=8  frac_width=24  explicit_period=on  period=ts*4  equ=P=C  opselect=C  inp2=PCIN>>17  opr=+  inp1=P  carry=CIN  dbl_ovrd=off  block_type=constant
  Convert : xbsIndex_r4/Convert  gui_display_data_type=Fixed-point  arith_type="Signed  (2's comp)"  n_bits=16  bin_pt=0  float_type=Single  exp_bits=8  fraction_bits=24  quantization="Round  (unbiased: +/- Inf)"  overflow=Saturate  en=off  latency=1  pipeline=off  dbl_ovrd=off  block_type=convert
  Convert1 : xbsIndex_r4/Convert  gui_display_data_type=Fixed-point  arith_type="Signed  (2's comp)"  n_bits=16  bin_pt=0  float_type=Single  exp_bits=8  fraction_bits=24  quantization="Round  (unbiased: +/- Inf)"  overflow=Saturate  en=off  latency=1  pipeline=off  dbl_ovrd=off  block_type=convert
  Terminator : Terminator
  data_out_im : Outport
  data_out_re : Outport  Port=2
  wires:
  Convert/1 -> data_out_im/1
  Convert1/1 -> data_out_re/1
  data_re/1 -> Complex Multiplier 6.0/3
  Constant3/1 -> Complex Multiplier 6.0/1
  Complex Multiplier 6.0/2 -> Convert/1
  Complex Multiplier 6.0/1 -> Terminator/1
  Constant1/1 -> Complex Multiplier 6.0/4
  sin/1 -> Complex Multiplier 6.0/5
  cosin/1 -> Complex Multiplier 6.0/6
  data_im/1 -> Complex Multiplier 6.0/2
  Complex Multiplier 6.0/3 -> Convert1/1

== system dsp_channelized_receiver_/fir_8path_ss/duc/duc_8line/CM7 ==
  data_re : Inport
  data_im : Inport  Port=2
  sin : Inport  Port=3
  cosin : Inport  Port=4
  Complex Multiplier 6.0 : xbsIndex_r4/Complex Multiplier 6.0   hasatlast=off  hasatuser=off  atuserwidth=1  hasbtlast=off  hasbtuser=off  btuserwidth=1  multtype=Use_Mults  optimizegoal=Performance  flowcontrol=NonBlocking  outputwidth=33  roundmode=Truncate  hasctrltlast=off  hasctrltuser=off  ctrltuserwidth=1  outtlastbehv=Null  latencyconfig=Automatic  minimumlatency=34  aclken=off  aresetn=off  trim_axipin_name=on  simulation_type=hybrid_sim  simulation_model=sysgen:cmpy_v6_0  data_path_portlist={ 's_axis_a_tdata_real', 's_axis_a_tdata_imag', 's_axis_b_tdata_real', 's_axis_b_tdata_imag', 's_axis_ctrl_tdata_rounding_bit', 'm_axis_dout_tdata_real', 'm_axis_dout_tdata_imag' }  aportwidth=63  bportwidth=63  ip_name=Complex Multiplier  ip_version=6.0  dsptool_ready=true  ipcore_usecache=true  ipcore_useipmodelcache=true  ipcore_verbose=false  ipcore_latency_parameter='minimumlatency'  wrapper_available=true  port_translation_map={ 'aclken' => 'en', 'aresetn' => 'rst'}  block_type=cmpy_v6_0
  Constant1 : xbsIndex_r4/Constant  const=1  gui_display_data_type=Boolean  arith_type=Boolean  n_bits=16  bin_pt=14  preci_type=Single  exp_width=8  frac_width=24  explicit_period=on  period=ts*4  equ=P=C  opselect=C  inp2=PCIN>>17  opr=+  inp1=P  carry=CIN  dbl_ovrd=off  block_type=constant
  Constant3 : xbsIndex_r4/Constant  const=1  gui_display_data_type=Boolean  arith_type=Boolean  n_bits=16  bin_pt=14  preci_type=Single  exp_width=8  frac_width=24  explicit_period=on  period=ts*4  equ=P=C  opselect=C  inp2=PCIN>>17  opr=+  inp1=P  carry=CIN  dbl_ovrd=off  block_type=constant
  Convert : xbsIndex_r4/Convert  gui_display_data_type=Fixed-point  arith_type="Signed  (2's comp)"  n_bits=16  bin_pt=0  float_type=Single  exp_bits=8  fraction_bits=24  quantization="Round  (unbiased: +/- Inf)"  overflow=Saturate  en=off  latency=1  pipeline=off  dbl_ovrd=off  block_type=convert
  Convert1 : xbsIndex_r4/Convert  gui_display_data_type=Fixed-point  arith_type="Signed  (2's comp)"  n_bits=16  bin_pt=0  float_type=Single  exp_bits=8  fraction_bits=24  quantization="Round  (unbiased: +/- Inf)"  overflow=Saturate  en=off  latency=1  pipeline=off  dbl_ovrd=off  block_type=convert
  Terminator : Terminator
  data_out_im : Outport
  data_out_re : Outport  Port=2
  wires:
  Complex Multiplier 6.0/3 -> Convert1/1
  data_im/1 -> Complex Multiplier 6.0/2
  cosin/1 -> Complex Multiplier 6.0/6
  sin/1 -> Complex Multiplier 6.0/5
  Constant1/1 -> Complex Multiplier 6.0/4
  Complex Multiplier 6.0/1 -> Terminator/1
  Complex Multiplier 6.0/2 -> Convert/1
  Constant3/1 -> Complex Multiplier 6.0/1
  data_re/1 -> Complex Multiplier 6.0/3
  Convert1/1 -> data_out_re/1
  Convert/1 -> data_out_im/1

== system dsp_channelized_receiver_/fir_8path_ss/duc/duc_8line/CM8 ==
  data_re : Inport
  data_im : Inport  Port=2
  sin : Inport  Port=3
  cosin : Inport  Port=4
  Complex Multiplier 6.0 : xbsIndex_r4/Complex Multiplier 6.0   hasatlast=off  hasatuser=off  atuserwidth=1  hasbtlast=off  hasbtuser=off  btuserwidth=1  multtype=Use_Mults  optimizegoal=Performance  flowcontrol=NonBlocking  outputwidth=33  roundmode=Truncate  hasctrltlast=off  hasctrltuser=off  ctrltuserwidth=1  outtlastbehv=Null  latencyconfig=Automatic  minimumlatency=34  aclken=off  aresetn=off  trim_axipin_name=on  simulation_type=hybrid_sim  simulation_model=sysgen:cmpy_v6_0  data_path_portlist={ 's_axis_a_tdata_real', 's_axis_a_tdata_imag', 's_axis_b_tdata_real', 's_axis_b_tdata_imag', 's_axis_ctrl_tdata_rounding_bit', 'm_axis_dout_tdata_real', 'm_axis_dout_tdata_imag' }  aportwidth=63  bportwidth=63  ip_name=Complex Multiplier  ip_version=6.0  dsptool_ready=true  ipcore_usecache=true  ipcore_useipmodelcache=true  ipcore_verbose=false  ipcore_latency_parameter='minimumlatency'  wrapper_available=true  port_translation_map={ 'aclken' => 'en', 'aresetn' => 'rst'}  block_type=cmpy_v6_0
  Constant1 : xbsIndex_r4/Constant  const=1  gui_display_data_type=Boolean  arith_type=Boolean  n_bits=16  bin_pt=14  preci_type=Single  exp_width=8  frac_width=24  explicit_period=on  period=ts*4  equ=P=C  opselect=C  inp2=PCIN>>17  opr=+  inp1=P  carry=CIN  dbl_ovrd=off  block_type=constant
  Constant3 : xbsIndex_r4/Constant  const=1  gui_display_data_type=Boolean  arith_type=Boolean  n_bits=16  bin_pt=14  preci_type=Single  exp_width=8  frac_width=24  explicit_period=on  period=ts*4  equ=P=C  opselect=C  inp2=PCIN>>17  opr=+  inp1=P  carry=CIN  dbl_ovrd=off  block_type=constant
  Convert : xbsIndex_r4/Convert  gui_display_data_type=Fixed-point  arith_type="Signed  (2's comp)"  n_bits=16  bin_pt=0  float_type=Single  exp_bits=8  fraction_bits=24  quantization="Round  (unbiased: +/- Inf)"  overflow=Saturate  en=off  latency=1  pipeline=off  dbl_ovrd=off  block_type=convert
  Convert1 : xbsIndex_r4/Convert  gui_display_data_type=Fixed-point  arith_type="Signed  (2's comp)"  n_bits=16  bin_pt=0  float_type=Single  exp_bits=8  fraction_bits=24  quantization="Round  (unbiased: +/- Inf)"  overflow=Saturate  en=off  latency=1  pipeline=off  dbl_ovrd=off  block_type=convert
  Terminator : Terminator
  data_out_im : Outport
  data_out_re : Outport  Port=2
  wires:
  Convert/1 -> data_out_im/1
  Convert1/1 -> data_out_re/1
  data_re/1 -> Complex Multiplier 6.0/3
  Constant3/1 -> Complex Multiplier 6.0/1
  Complex Multiplier 6.0/2 -> Convert/1
  Complex Multiplier 6.0/1 -> Terminator/1
  Constant1/1 -> Complex Multiplier 6.0/4
  sin/1 -> Complex Multiplier 6.0/5
  cosin/1 -> Complex Multiplier 6.0/6
  data_im/1 -> Complex Multiplier 6.0/2
  Complex Multiplier 6.0/3 -> Convert1/1
